simulink model "sgMdl_IO130_DMALoopback"  (R2024b)
settings: Solver=FixedStepAuto  StartTime=0.0  StopTime=inf  RelTol=1e-3  EnableMultiTasking=on
libraries: speedgoatlib_IO130 x3, speedgoatlib_interrupt x1, dspsrcs4 x1
Description:
  | IO130 - DMA Loopback
settings Model: sg_rtwmakecfg_data=_sglibc_  ModifiedByFormat=Speedgoat  Creator=Speedgoat  LastModifiedBy=Speedgoat
settings SolverCC: ConcurrentTasks=on  AlgebraicLoopSolver=TrustRegion  PositivePriorityOrder=on  AutoInsertRateTranBlk=on  InsertRTBMode=Never (minimum delay)
settings DataIOCC: SaveFormat=StructureWithTime  ReturnWorkspaceOutputs=off
settings OptimizationCC: BlockReduction=off  OptimizeBlockIOStorage=off  BufferReuse=off  GlobalBufferReuse=off  ExpressionFolding=off  LocalBlockOutputs=off
settings DebuggingCC: TasksWithSamePriorityMsg=none  UnconnectedInputMsg=warning  UnconnectedOutputMsg=warning  UnconnectedLineMsg=warning  SFExecutionAtInitializationDiag=none  ArithmeticOperatorsInVariantConditions=warning
settings HardwareCC: ProdBitPerLong=64  ProdLongLongMode=on  ProdHWDeviceType=Intel->x86-64 (Linux 64)
settings ModelReferenceCC: EnableRefExpFcnMdlSchedulingChecks=on
settings SFSimCC: SimUseLocalCustomCode=off  CustomCodeUndefinedFunction=UseInterfaceOnly
settings RTWCC: Description=Speedgoat Real-Time Target Machine  SystemTargetFile=speedgoat.tlc  TemplateMakefile=slrealtime_default_tmf  RTWUseLocalCustomCode=off  Toolchain=Simulink Real-Time Toolchain  BuildConfiguration=Faster Runs  TargetLang=C++  GPUComputeCapability=3.5  DLArmComputeVersion=19.05
settings CodeAppCC: StateflowObjectComments=on
settings SimulinkRealTimeTargetCC: SubcomponentCodeInterfacePackaging=Reusable function  InstructionSetFMA=off  LogToMDFFile=off  SLRTFileLogMaxRuns=10  UseGCCFastMath=on
settings ConfigComp: CovBoundaryAbsTol=1.0e-5

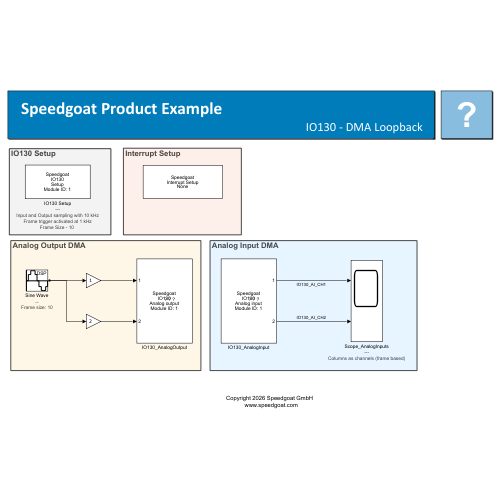
[thumbnail: Simulink's stored preview of the top-level diagram]
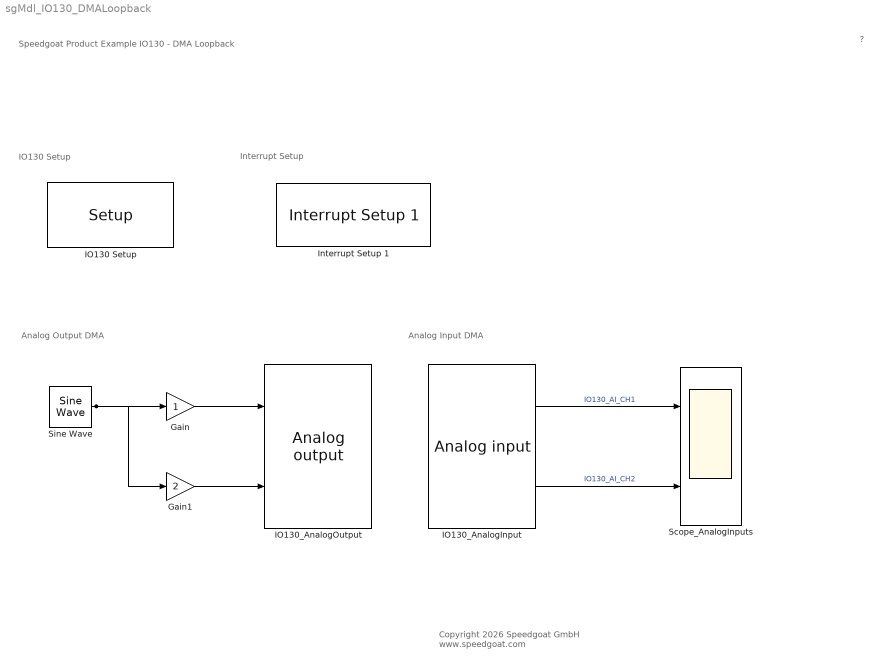
== system sgMdl_IO130_DMALoopback ==
  note: Analog Output DMA
  note: Analog Input DMA
  note: Interrupt Setup
  note: IO130 Setup
  note: Speedgoat Product Example
      | IO130 - DMA Loopback
  note: ?
  note: Copyright 2026 Speedgoat GmbH
      |  www.speedgoat.com
  Gain : Gain
  Gain1 : Gain  Gain=2
  IO130 Setup : speedgoatlib_IO130/Setup   parPciSlot=-1  parModuleId=1  parTriggerInitiator=Independent  parAdChannels=[1 2]  parAdRange=+-10V  parAdOversampling=None  parAdContinuousSampling=off  parAdDmaEn=on  parAdDisableCheck=off  parAdDmaChannels=All  parAdSampleClock=10e3  parAdDmaFrameSize=10  parAdSampleTime=-1  parDaChannels=[1 2]  parDaRange=+-10V  parDaInitValues=[0]  parDaResetValues=[1]  parDaDmaEn=on  parDaDisableCheck=off  parDaDmaChannels=All  parLatency=As small as possible  parDaSampleClock=10e3  parClockLocked=on  parDaDmaFrameSize=10  parDaSampleTime=-1  parBoardType=130  parForceRefresh=11[]
      settings: SourceProductName=Simulink Real-Time: Speedgoat Library
      settings: AttributesFormatString=|
      | ---
      | Input and Output sampling with 10 kHz
      | Frame trigger activated at 1 kHz
      | Frame Size - 10
  IO130_AnalogInput : speedgoatlib_IO130/Analog input   parModuleId=1  parSampleTime=0.001  parPciSlot=-1  parRange=+-10V  parOversampling=None  parChannels=[1 2]  parContinuousSampling=off  parDmaEn=on  parDmaChannels=All  parDmaConversionTime=1000  parDmaFrameSize=10  parBoardType=130  parIsInitialized=on
      settings: SourceProductName=Simulink Real-Time: Speedgoat Library
  IO130_AnalogOutput : speedgoatlib_IO130/Analog output   parModuleId=1  parSampleTime=0.001  parPciSlot=-1  parRange=+-10V  parChannels=[1 2]  parInitValues=[0 0]  parResetValues=[1 1]  parDmaChannels=All  parDmaEn=on  parDmaClkSrc=2  parDmaConversionTime=1000  parDmaFrameSize=10  parBoardType=130  parDoInterrupt=off  parLatency=As small as possible  parIsInitialized=on
      settings: SourceProductName=Simulink Real-Time: Speedgoat Library
  Interrupt Setup 1 : speedgoatlib_interrupt/Interrupt Setup 1  parModuleTrigger=on  parPollingMode=off  parPriorityConf=High  parPriority=241  confStartFcn=IO130_start_public  confStopFcn=IO130_stop_public  confIsrFcn=IO130_isr_public  confMapFcn=IO130_map_public  confHookFile=io130_int_hooks.c  confIrqNr=-1  confIsPolling=off  confModID=16776961  confSelectedInt=Speedgoat IO130 DMA interrupt  confSelectedId=1  confSelectedChannel=[]  confData=[]  confForcePollingMode=off
  Scope_AnalogInputs : Scope  NumInputPorts=2
      settings: AttributesFormatString=|
      | ---
      | %<FrameBasedProcessingString>
  Sine Wave : dspsrcs4/Sine Wave  Amplitude=1  Frequency=100  Phase=0  SampleMode=Discrete  OutComplex=Real  CompMethod=Trigonometric fcn  TableSize=Speed  SampleTime=1/10000  SamplesPerFrame=10  ResetState=Restart at time zero  OutputFrames=off  dataType=double  wordLen=16  udDataType=sfix(16)  fracBitsMode=Best precision  numFracBits=15  OutDataTypeStr=double  LastOutDataTypeStr=double
      settings: AttributesFormatString=|
      | --
      | Frame size: %<SamplesPerFrame>
  wires:
  Sine Wave/1 -> Gain1/1, Gain/1
  Gain/1 -> IO130_AnalogOutput/1
  Gain1/1 -> IO130_AnalogOutput/2
  IO130_AnalogInput/2 -> Scope_AnalogInputs/2  "IO130_AI_CH2"
  IO130_AnalogInput/1 -> Scope_AnalogInputs/1  "IO130_AI_CH1"
